simulink model "main"  (R2025b)
settings: Solver=FixedStepDiscrete  StartTime=0.0  StopTime=Inf  RelTol=1e-3  EnableMultiTasking=on
PreLoadFcn:
  | RTWConfigurationCB('preloadfcn', bdroot);
model workspace (MAT data in the model file):
  fault_count = 0
  fz_values = [0 50 100 150 200 250 300 350 400 450 500 550 ... (43 elements, 1x43)]
  k_opt_lut = [0 0 0 0 0 0 0 0 0 0 0 0 ... (4386 elements, 51x2x43)]
  mu_opt_lut = [0 0 0 0 0 0 0 0 0 0 0 0 ... (4386 elements, 51x2x43)]
undefined symbols (not defined in the file or in its folder): bit, Call, Function, ocv_lut, slope_lut, soc_lut
libraries: c2837xDlib x34, c280xlib x20, canmsglib x18, c2802xlib x12, simulink x9, slpidlib x3
(part 3 of 5)

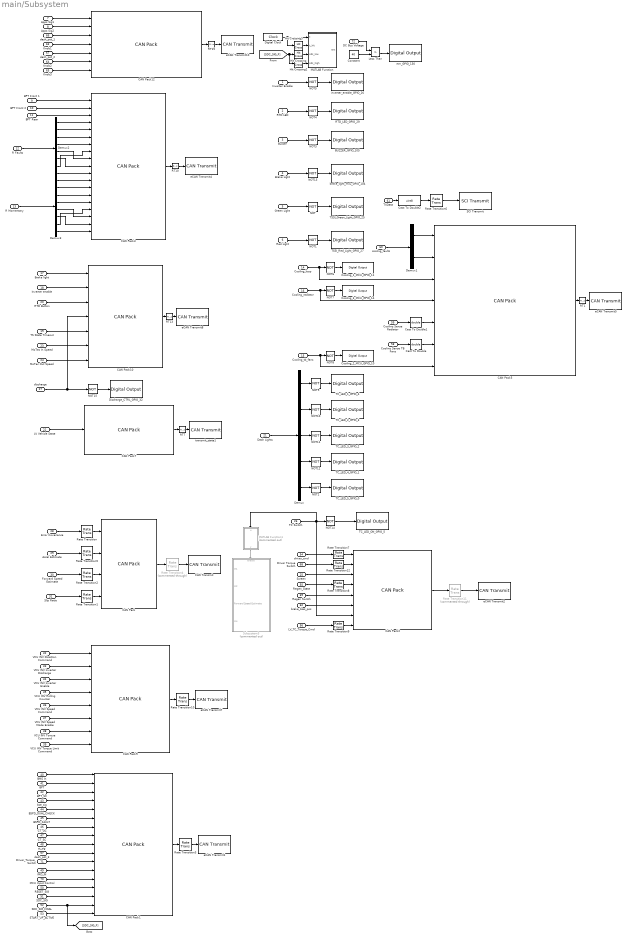
== system main/Subsystem ==
  Inverter Enable : Inport
  RTD LED : Inport  Port=2
  Buzzer : Inport  Port=3
  Brake Light : Inport  Port=4
  Green Light : Inport  Port=5
  Red Light : Inport  Port=6
  Apps Sig1 : Inport  Port=7
  Apps Sig2 : Inport  Port=8
  BPT Front 1 : Inport  Port=9
  BPT Front 2 : Inport  Port=10
  BPT Rear : Inport  Port=11
  R Faults : Inport  Port=12
  R Momentary : Inport  Port=13
  Cooling_loop : Inport  Port=14
  Cooling_tb_fans : Inport  Port=15
  Cooling_radiator : Inport  Port=16
  Brake light : Inport  Port=17
  Inverter enable : Inport  Port=18
  TS State Timeout : Inport  Port=19
  RTD Button : Inport  Port=20
  Dash Lights : Inport  Port=21
  LV Vehicle State : Inport  Port=22
  MoTec In Speed : Inport  Port=23
  MoTec Out Speed : Inport  Port=24
  Screen : Inport  Port=25
  TC Switch : Inport  Port=26
  discharge : Inport  Port=27
  Error Covariance : Inport  Port=28
  Accel Estimate : Inport  Port=29
  Forward Speed Estimate : Inport  Port=30
  Slip Ratio : Inport  Port=31
  VCU INV Direction Command : Inport  Port=32
  VCU INV Inverter Discharge : Inport  Port=33
  VCU INV Inverter Enable : Inport  Port=34
  VCU INV Rolling Counter : Inport  Port=35
  VCU INV Speed Command : Inport  Port=36
  VCU INV Speed Mode Enable : Inport  Port=37
  VCU INV Torque Command : Inport  Port=38
  VCU INV Torque Limit Command : Inport  Port=39
  BMS In : Inport  Port=40
  BPT : Inport  Port=41
  BPT_SC : Inport  Port=42
  bse_sig : Inport  Port=43
  BSPD_DUAL_CHECK : Inport  Port=44
  BSPD_FAULT : Inport  Port=45
  CT_OC : Inport  Port=46
  CT_SC : Inport  Port=47
  ct_sig : Inport  Port=48
  IMD_IN : Inport  Port=49
  RESET_SIG : Inport  Port=50
  SDC_SIG : Inport  Port=51
  SDC_SIG_FINAL : Inport  Port=52
  START_UP_ACTIVE : Inport  Port=53
  driver_cmd : Inport  Port=54
  Regen_State : Inport  Port=55
  LV_TC_Torque_Cmd : Inport  Port=56
  dash_pot_3 : Inport  Port=57
  Cooling Sense TB Fans : Inport  Port=58
  Cooling Sense Radiator : Inport  Port=59
  cooling_faults : Inport  Port=60
  TXData : Inport  Port=61
  brake_bias_pos : Inport  Port=62
  Knob1 : Inport  Port=63
  Knob2 : Inport  Port=64
  Knob3 : Inport  Port=65
  dash_pot_1 : Inport  Port=66
  dash_pot_2 : Inport  Port=67
  Driver Torque Switch : Inport  Port=68
  Regen Switch : Inport  Port=69
  MCU Input Control : Inport  Port=70
  Driver_Torque_Switch : Inport  Port=71
  DC Bus Voltage : Inport  Port=72
  BUZZER_GPIO_105 : c2837xDlib/Digital Output  GPIO_Number=GPIO104~GPIO111  GPIO_Bit0=off  GPIO_BIT0_Toggle=off  GPIO_Bit1=on  GPIO_BIT1_Toggle=off  GPIO_Bit2=off  GPIO_BIT2_Toggle=off  GPIO_Bit3=off  GPIO_BIT3_Toggle=off  GPIO_Bit4=off  GPIO_BIT4_Toggle=off  GPIO_Bit5=off  GPIO_BIT5_Toggle=off  GPIO_Bit6=off  GPIO_BIT6_Toggle=off  GPIO_Bit7=off  GPIO_BIT7_Toggle=off
  CAN Pack : canmsglib/CAN Pack  CANdbFile=C:\Users\Columbia\Documents\GitHub\EV26-Software\CAN\EV26.dbc  MsgList=(none)  MsgName=M404_LV_V_Kalman_Outputs  MsgIDType=Standard (11-bit identifier)  MsgIdentifier=404  CANIDInput=off  MsgLength=8  Remote=off  ApplyMinMax=off  BusOutput=off  SignalInfo={'LV_COV_V','32','16','LE','unsigned','Standard','0','0.02','0','0','1310.7';'LV_FILTERED_A','16','16','LE','signed','Standard','0','0.01','0','-327.68','327.67';'LV_FILTERED_V','0','16','LE','unsigned','Standard','0','0.1','0','0','6553.5';'LV_SR','48','16','LE','signed','Standard','0','0.0001','0','-3.2768','3.2767'}
      settings: LibrarySourceBlock=c2000lib/Target Communication/CAN Pack  DataFormat=CANdb specified signals
  CAN Pack1 : canmsglib/CAN Pack  CANdbFile=C:\Users\levin\OneDrive\Documents\GitHub\EV26-Software\CAN\EV26.dbc  MsgList=M406_Board_Signals  MsgName=M406_Board_Signals  MsgIDType=Standard (11-bit identifier)  MsgIdentifier=406  CANIDInput=off  MsgLength=8  Remote=off  ApplyMinMax=off  BusOutput=off  SignalInfo={'LV_BMS_Good','1','1','LE','unsigned','Standard','0','1','0','0','1';'LV_BPT_OC','3','1','LE','unsigned','Standard','0','1','0','0','1';'LV_BPT_SC','2','1','LE','unsigned','Standard','0','1','0','0','1';'LV_BSE_Sig','16','16','LE','signed','Standard','0','1','0','-32768','32767';'LV_BSPD_Dual_Check','6','1','LE','unsigned','Standard','0','1','0','0','1';'LV_BSPD_Fault','7','1','LE','unsigned','Standard','0','1','0','0','1';'LV_CT_OC','5','1','LE','unsigned','Standard','0','1','0','0','1';'LV_CT_SC','4','1','LE','unsigned','Standard','0','1','0','0','1';'LV_CT_Sig','32','16','LE','signed','Standard','0','1','0','-32768','32767';'LV_Dash_Pot_3','48','8','LE','unsigned','Standard','0','20','0','0','5100';'LV_Driver_Torque_Switch','56','1','LE','unsigned','Standard','0','1','0','0','1';'LV_IMD_Good','0','1','LE','unsigned','Standard','0','1','0','0','1';'LV_MCU_Torque_Ctrl','12','3','LE','unsigned','Standard','0','1','0','0','7';'LV_Reset_Sig','10','1','LE','unsigned','Standard','0','1','0','0','1';'LV_SDC_Sig','11','1','LE','unsigned','Standard','0','1','0','0','1';'LV_SDC_Sig_Final','9','1','LE','unsigned','Standard','0','1','0','0','1';'LV_Start_Up_Active','8','1','LE','unsigned','Standard','0','1','0','0','1'}
      settings: DataFormat=CANdb specified signals
  CAN Pack10 : canmsglib/CAN Pack  CANdbFile=C:\Users\levin\OneDrive\Documents\GitHub\EV26-Software\CAN\EV26.dbc  MsgList=M403_Vehicle_State_Inputs  MsgName=M403_Vehicle_State_Inputs  MsgIDType=Standard (11-bit identifier)  MsgIdentifier=403  CANIDInput=off  MsgLength=8  Remote=off  ApplyMinMax=off  BusOutput=off  SignalInfo={'LV_Brake_Light','0','8','LE','unsigned','Standard','0','1','0','-Inf','Inf';'LV_Echo_Inverter_Enable','8','8','LE','signed','Standard','0','1','0','-Inf','Inf';'LV_RTD_Button','24','8','LE','unsigned','Standard','0','1','0','-Inf','Inf';'LV_TB_Discharge','32','1','LE','unsigned','Standard','0','1','0','0','1';'LV_TB_TS_State_Timeout','16','8','LE','signed','Standard','0','1','0','-Inf','Inf';'MoTec_In_Speed','40','12','LE','unsigned','Standard','0','0.1','0','0','409.5';'MoTec_Out_Speed','52','12','LE','unsigned','Standard','0','0.1','0','0','409.5'}
      settings: DataFormat=CANdb specified signals
  CAN Pack12 : canmsglib/CAN Pack  CANdbFile=C:\Users\levin\OneDrive\Documents\GitHub\EV26-Software\CAN\EV26.dbc  MsgList=M401_Accelerator_Controls  MsgName=M401_Accelerator_Controls  MsgIDType=Standard (11-bit identifier)  MsgIdentifier=401  CANIDInput=off  MsgLength=8  Remote=off  ApplyMinMax=off  BusOutput=off  SignalInfo={'LV_APPS1','0','16','LE','unsigned','Standard','0','1','0','0','4095';'LV_APPS2','16','16','LE','unsigned','Standard','0','1','0','0','4095';'LV_Dash_Pot_1','44','8','LE','unsigned','Standard','0','20','0','0','5100';'LV_Dash_Pot_1_Tick','32','4','LE','unsigned','Standard','0','1','0','0','15';'LV_Dash_Pot_2','52','8','LE','unsigned','Standard','0','20','0','0','5100';'LV_Dash_Pot_2_Tick','36','4','LE','unsigned','Standard','0','1','0','0','15';'LV_Dash_Pot_3_Tick','40','4','LE','unsigned','Standard','0','1','0','0','15'}
      settings: DataFormat=CANdb specified signals
  CAN Pack2 : canmsglib/CAN Pack  CANdbFile=C:\Users\levin\OneDrive\Documents\GitHub\EV26-Software\CAN\EV26.dbc  MsgList=M405_TC_Regen_Signals  MsgName=M405_TC_Regen_Signals  MsgIDType=Standard (11-bit identifier)  MsgIdentifier=405  CANIDInput=off  MsgLength=8  Remote=off  ApplyMinMax=off  BusOutput=off  SignalInfo={'LV_Driver_Torque','16','16','LE','signed','Standard','0','0.1','0','-3276.8','3276.7';'LV_Driver_Torque_Switch','58','1','LE','unsigned','Standard','0','1','0','0','1';'LV_MoTec_Screen','48','8','LE','unsigned','Standard','0','1','0','0','255';'LV_Regen_State','32','8','LE','signed','Standard','0','1','0','-128','127';'LV_Regen_Switch','57','1','LE','unsigned','Standard','0','1','0','0','1';'LV_Servo_Pos','40','8','LE','signed','Standard','0','160.6275','0','-20560.3137','20399.6863';'LV_TC_Switch','56','1','LE','unsigned','Standard','0','1','0','0','1';'LV_TC_Torque_Cmd','0','16','LE','signed','Standard','0','0.1','0','-3276.8','3276.7'}
      settings: DataFormat=CANdb specified signals
  CAN Pack3 : canmsglib/CAN Pack  CANdbFile=C:\Users\Columbia\Documents\GitHub\EV26-Software\CAN\EV26.dbc  MsgList=(none)  MsgName=M402_Brakes_Faults_Display  MsgIDType=Standard (11-bit identifier)  MsgIdentifier=402  CANIDInput=off  MsgLength=8  Remote=off  ApplyMinMax=off  BusOutput=off  SignalInfo={'LV_BPT_Front_1','16','16','LE','unsigned','Standard','0','1','0','-Inf','Inf';'LV_BPT_Front_2','32','16','LE','unsigned','Standard','0','1','0','-Inf','Inf';'LV_BPT_Rear','0','16','LE','unsigned','Standard','0','1','0','-Inf','Inf';'LV_Fault_APPS1_Lower','48','1','LE','unsigned','Standard','0','1','0','0','1';'LV_Fault_APPS1_Upper','49','1','LE','unsigned','Standard','0','1','0','0','1';'LV_Fault_APPS2_Lower','50','1','LE','unsigned','Standard','0','1','0','0','1';'LV_Fault_APPS2_Upper','51','1','LE','unsigned','Standard','0','1','0','0','1';'LV_Fault_APPS_Implausibility','54','1','LE','unsigned','Standard','0','1','0','0','1';'LV_Fault_BPT_Lower','52','1','LE','unsigned','Standard','0','1','0','0','1';'LV_Fault_BPT_Upper','53','1','LE','unsigned','Standard','0','1','0','0','1';'LV_Fault_Both_Pedals','55','1','LE','unsigned','Standard','0','1','0','0','1';'LV_Momentary_APPS1_Lower','56','1','LE','unsigned','Standard','0','1','0','0','1';'LV_Momentary_APPS1_Upper','57','1','LE','unsigned','Standard','0','1','0','0','1';'LV_Momentary_APPS2_Lower','58','1','LE','unsigned','Standard','0','1','0','0','1';'LV_Momentary_APPS2_Upper','59','1','LE','unsigned','Standard','0','1','0','0','1';'LV_Momentary_APPS_Implausibility','62','1','LE','unsigned','Standard','0','1','0','0','1';'LV_Momentary_BPT_Lower','60','1','LE','unsigned','Standard','0','1','0','0','1';'LV_Momentary_BPT_Upper','61','1','LE','unsigned','Standard','0','1','0','0','1';'LV_Momentary_Both_Pedals','63','1','LE','unsigned','Standard','0','1','0','0','1'}
      settings: DataFormat=CANdb specified signals
  CAN Pack5 : canmsglib/CAN Pack  CANdbFile=C:\Users\levin\OneDrive\Documents\GitHub\EV26-Software\CAN\EV26.dbc  MsgList=M003_DCDC_Enable_Cooling  MsgName=M003_DCDC_Enable_Cooling  MsgIDType=Standard (11-bit identifier)  MsgIdentifier=3  CANIDInput=off  MsgLength=8  Remote=off  ApplyMinMax=off  BusOutput=off  SignalInfo={'LV_TB_Cooling_Fault_Radiator','36','1','LE','unsigned','Standard','0','1','0','0','1';'LV_TB_Cooling_Fault_TB_Fans','35','1','LE','unsigned','Standard','0','1','0','0','1';'LV_TB_Cooling_Loop','32','1','LE','unsigned','Standard','0','1','0','0','1';'LV_TB_Cooling_Radiator','34','1','LE','unsigned','Standard','0','1','0','0','1';'LV_TB_Cooling_Sense_Radiator','16','16','LE','signed','Standard','0','0.01','0','-327.68','327.67';'LV_TB_Cooling_Sense_TB_Fans','0','16','LE','signed','Standard','0','0.01','0','-327.68','327.67';'LV_TB_Cooling_TB_Fans','33','1','LE','unsigned','Standard','0','1','0','0','1'}
      settings: DataFormat=CANdb specified signals
  CAN Pack7 : canmsglib/CAN Pack  CANdbFile=C:\Users\Columbia\Documents\GitHub\EV26-Software\CAN\EV26.dbc  MsgList=(none)  MsgName=M001_Vehicle_State  MsgIDType=Standard (11-bit identifier)  MsgIdentifier=1  CANIDInput=off  MsgLength=1  Remote=off  ApplyMinMax=off  BusOutput=off  SignalInfo={'LV_Vehicle_State','0','8','LE','signed','Standard','0','1','0','-Inf','Inf'}
      settings: DataFormat=CANdb specified signals
  CAN Pack9 : canmsglib/CAN Pack  CANdbFile=C:\Users\levin\OneDrive\Documents\GitHub\EV26-Software\CAN\EV26.dbc  MsgList=M192_Command_Message  MsgName=M192_Command_Message  MsgIDType=Standard (11-bit identifier)  MsgIdentifier=192  CANIDInput=off  MsgLength=8  Remote=off  ApplyMinMax=off  BusOutput=off  SignalInfo={'VCU_INV_Direction_Command','32','1','LE','unsigned','Standard','0','1','0','0','1';'VCU_INV_Inverter_Discharge','41','1','LE','unsigned','Standard','0','1','0','0','1';'VCU_INV_Inverter_Enable','40','1','LE','unsigned','Standard','0','1','0','0','1';'VCU_INV_Rolling_Counter','44','4','LE','unsigned','Standard','0','1','0','0','15';'VCU_INV_Speed_Command','16','16','LE','signed','Standard','0','1','0','-32768','32767';'VCU_INV_Speed_Mode_Enable','42','1','LE','unsigned','Standard','0','1','0','0','1';'VCU_INV_Torque_Command','0','16','LE','signed','Standard','0','0.1','0','-3276.8','3276.7';'VCU_INV_Torque_Limit_Command','48','16','LE','signed','Standard','0','0.1','0','-3276.8','3276.7'}
      settings: DataFormat=CANdb specified signals
  CAN Transmit : c280xlib/CAN Transmit  chipFamily=C280x  useModule=CAN_B  mailboxNo=11  messageID=404  messageType=Standard (11-bit identifier)  enableBlockingMode=off  postInterrupt=off  interruptLine=0
  Cast To Double : DataTypeConversion  OutDataTypeStr=double  SaturateOnIntegerOverflow=off  RndMeth=Floor
  Cast To Double1 : DataTypeConversion  OutDataTypeStr=double  SaturateOnIntegerOverflow=off  RndMeth=Floor
  Cast To Double2 : DataTypeConversion  OutDataTypeStr=uint8  SaturateOnIntegerOverflow=off  RndMeth=Floor
  Constant : Constant  Value=40
  Cooling_1_MCU_GPIO_11 : c2837xDlib/Digital Output  GPIO_Number=GPIO8~GPIO15  GPIO_Bit0=off  GPIO_BIT0_Toggle=off  GPIO_Bit1=off  GPIO_BIT1_Toggle=off  GPIO_Bit2=off  GPIO_BIT2_Toggle=off  GPIO_Bit3=on  GPIO_BIT3_Toggle=off  GPIO_Bit4=off  GPIO_BIT4_Toggle=off  GPIO_Bit5=off  GPIO_BIT5_Toggle=off  GPIO_Bit6=off  GPIO_BIT6_Toggle=off  GPIO_Bit7=off  GPIO_BIT7_Toggle=off
  Cooling_2_MCU_GPIO_10 : c2837xDlib/Digital Output  GPIO_Number=GPIO8~GPIO15  GPIO_Bit0=off  GPIO_BIT0_Toggle=off  GPIO_Bit1=off  GPIO_BIT1_Toggle=off  GPIO_Bit2=on  GPIO_BIT2_Toggle=off  GPIO_Bit3=off  GPIO_BIT3_Toggle=off  GPIO_Bit4=off  GPIO_BIT4_Toggle=off  GPIO_Bit5=off  GPIO_BIT5_Toggle=off  GPIO_Bit6=off  GPIO_BIT6_Toggle=off  GPIO_Bit7=off  GPIO_BIT7_Toggle=off
  Cooling_3_MCU_GPIO_14 : c2837xDlib/Digital Output  GPIO_Number=GPIO8~GPIO15  GPIO_Bit0=off  GPIO_BIT0_Toggle=off  GPIO_Bit1=off  GPIO_BIT1_Toggle=off  GPIO_Bit2=off  GPIO_BIT2_Toggle=off  GPIO_Bit3=off  GPIO_BIT3_Toggle=off  GPIO_Bit4=off  GPIO_BIT4_Toggle=off  GPIO_Bit5=off  GPIO_BIT5_Toggle=off  GPIO_Bit6=on  GPIO_BIT6_Toggle=off  GPIO_Bit7=off  GPIO_BIT7_Toggle=off
  Demux : Demux  Outputs=5
  Demux1 : Demux  Outputs=2
  Demux2 : Demux  Outputs=8
  Demux3 : Demux  Outputs=8
  Digital Clock : DigitalClock  SampleTime=0.001
  Discharge_CTRL_GPIO_32 : c2837xDlib/Digital Output  GPIO_Number=GPIO32~GPIO39  GPIO_Bit0=on  GPIO_BIT0_Toggle=off  GPIO_Bit1=off  GPIO_BIT1_Toggle=off  GPIO_Bit2=off  GPIO_BIT2_Toggle=off  GPIO_Bit3=off  GPIO_BIT3_Toggle=off  GPIO_Bit4=off  GPIO_BIT4_Toggle=off  GPIO_Bit5=off  GPIO_BIT5_Toggle=off  GPIO_Bit6=off  GPIO_BIT6_Toggle=off  GPIO_Bit7=off  GPIO_BIT7_Toggle=off
  Hit Crossing : HitCross  HitCrossingDirection=falling
  Hit Crossing2 : HitCross  HitCrossingOffset=1  HitCrossingDirection=rising
  Hit Crossing3 : HitCross  HitCrossingOffset=4  HitCrossingDirection=rising
  Less Than : RelationalOperator  Operator=>  OutDataTypeStr=boolean  RndMeth=Simplest  InputSameDT=off
  MATLAB Function : MATLAB Function  TreatAsAtomicUnit=on
  MATLAB Function1 : MATLAB Function  Commented=on  TreatAsAtomicUnit=on
  NOT{,1..15} (16 alike) : Logic  Operator=NOT  IconShape=distinctive  AllPortsSameDT=off  OutDataTypeStr=boolean
  RT1 : RateTransition  OutPortSampleTime=.1
  RT10 : RateTransition  OutPortSampleTime=.01
  RT13 : RateTransition  OutPortSampleTime=.05
  RT15 : RateTransition  OutPortSampleTime=0.01
  RT7 : RateTransition  OutPortSampleTime=.1
  RTD_LED_GPIO_29 : c2837xDlib/Digital Output  GPIO_Number=GPIO24~GPIO31  GPIO_Bit0=off  GPIO_BIT0_Toggle=off  GPIO_Bit1=off  GPIO_BIT1_Toggle=off  GPIO_Bit2=off  GPIO_BIT2_Toggle=off  GPIO_Bit3=off  GPIO_BIT3_Toggle=off  GPIO_Bit4=off  GPIO_BIT4_Toggle=off  GPIO_Bit5=on  GPIO_BIT5_Toggle=off  GPIO_Bit6=off  GPIO_BIT6_Toggle=off  GPIO_Bit7=off  GPIO_BIT7_Toggle=off
  Rate Transition{,1..3,5,7..9,12} (9 alike) : RateTransition  OutPortSampleTime=0.01
  Rate Transition10 : RateTransition  OutPortSampleTime=0.003
  Rate Transition11 : RateTransition  Commented=through  OutPortSampleTime=0.003
  Rate Transition4 : RateTransition  Commented=through  OutPortSampleTime=0.05
  Rate Transition6 : RateTransition  OutPortSampleTime=1
  SCI Transmit : c280xlib/SCI Transmit  sciModule=C  dataHead='S'  dataTail='E'  frameSize=1  blockingMode=on  outputStatus=off
      settings: LibrarySourceBlock=c2802xlib/SCI Transmit
  Subsystem3 : Subsystem  Commented=on
  TC_LED_1_GPIO_4 : c2837xDlib/Digital Output  GPIO_Number=GPIO0~GPIO7  GPIO_Bit0=off  GPIO_BIT0_Toggle=off  GPIO_Bit1=off  GPIO_BIT1_Toggle=off  GPIO_Bit2=off  GPIO_BIT2_Toggle=off  GPIO_Bit3=off  GPIO_BIT3_Toggle=off  GPIO_Bit4=on  GPIO_BIT4_Toggle=off  GPIO_Bit5=off  GPIO_BIT5_Toggle=off  GPIO_Bit6=off  GPIO_BIT6_Toggle=off  GPIO_Bit7=off  GPIO_BIT7_Toggle=off
  TC_LED_2_GPIO_3 : c2837xDlib/Digital Output  GPIO_Number=GPIO0~GPIO7  GPIO_Bit0=off  GPIO_BIT0_Toggle=off  GPIO_Bit1=off  GPIO_BIT1_Toggle=off  GPIO_Bit2=off  GPIO_BIT2_Toggle=off  GPIO_Bit3=on  GPIO_BIT3_Toggle=off  GPIO_Bit4=off  GPIO_BIT4_Toggle=off  GPIO_Bit5=off  GPIO_BIT5_Toggle=off  GPIO_Bit6=off  GPIO_BIT6_Toggle=off  GPIO_Bit7=off  GPIO_BIT7_Toggle=off
  TC_LED_3_GPIO_2 : c2837xDlib/Digital Output  GPIO_Number=GPIO0~GPIO7  GPIO_Bit0=off  GPIO_BIT0_Toggle=off  GPIO_Bit1=off  GPIO_BIT1_Toggle=off  GPIO_Bit2=on  GPIO_BIT2_Toggle=off  GPIO_Bit3=off  GPIO_BIT3_Toggle=off  GPIO_Bit4=off  GPIO_BIT4_Toggle=off  GPIO_Bit5=off  GPIO_BIT5_Toggle=off  GPIO_Bit6=off  GPIO_BIT6_Toggle=off  GPIO_Bit7=off  GPIO_BIT7_Toggle=off
  TC_LED_4_GPIO_1 : c2837xDlib/Digital Output  GPIO_Number=GPIO0~GPIO7  GPIO_Bit0=off  GPIO_BIT0_Toggle=off  GPIO_Bit1=on  GPIO_BIT1_Toggle=off  GPIO_Bit2=off  GPIO_BIT2_Toggle=off  GPIO_Bit3=off  GPIO_BIT3_Toggle=off  GPIO_Bit4=off  GPIO_BIT4_Toggle=off  GPIO_Bit5=off  GPIO_BIT5_Toggle=off  GPIO_Bit6=off  GPIO_BIT6_Toggle=off  GPIO_Bit7=off  GPIO_BIT7_Toggle=off
  TC_LED_5_GPIO_0 : c2837xDlib/Digital Output  GPIO_Number=GPIO0~GPIO7  GPIO_Bit0=on  GPIO_BIT0_Toggle=off  GPIO_Bit1=off  GPIO_BIT1_Toggle=off  GPIO_Bit2=off  GPIO_BIT2_Toggle=off  GPIO_Bit3=off  GPIO_BIT3_Toggle=off  GPIO_Bit4=off  GPIO_BIT4_Toggle=off  GPIO_Bit5=off  GPIO_BIT5_Toggle=off  GPIO_Bit6=off  GPIO_BIT6_Toggle=off  GPIO_Bit7=off  GPIO_BIT7_Toggle=off
  TC_LED_ON_GPIO_5 : c2837xDlib/Digital Output  GPIO_Number=GPIO0~GPIO7  GPIO_Bit0=off  GPIO_BIT0_Toggle=off  GPIO_Bit1=off  GPIO_BIT1_Toggle=off  GPIO_Bit2=off  GPIO_BIT2_Toggle=off  GPIO_Bit3=off  GPIO_BIT3_Toggle=off  GPIO_Bit4=off  GPIO_BIT4_Toggle=off  GPIO_Bit5=on  GPIO_BIT5_Toggle=off  GPIO_Bit6=off  GPIO_BIT6_Toggle=off  GPIO_Bit7=off  GPIO_BIT7_Toggle=off
  TSSI_Green_Light_GPIO_25 : c2837xDlib/Digital Output  GPIO_Number=GPIO24~GPIO31  GPIO_Bit0=off  GPIO_BIT0_Toggle=off  GPIO_Bit1=on  GPIO_BIT1_Toggle=off  GPIO_Bit2=off  GPIO_BIT2_Toggle=off  GPIO_Bit3=off  GPIO_BIT3_Toggle=off  GPIO_Bit4=off  GPIO_BIT4_Toggle=off  GPIO_Bit5=off  GPIO_BIT5_Toggle=off  GPIO_Bit6=off  GPIO_BIT6_Toggle=off  GPIO_Bit7=off  GPIO_BIT7_Toggle=off
  TSSI_Red_Light_GPIO_27 : c2837xDlib/Digital Output  GPIO_Number=GPIO24~GPIO31  GPIO_Bit0=off  GPIO_BIT0_Toggle=off  GPIO_Bit1=off  GPIO_BIT1_Toggle=off  GPIO_Bit2=off  GPIO_BIT2_Toggle=off  GPIO_Bit3=on  GPIO_BIT3_Toggle=off  GPIO_Bit4=off  GPIO_BIT4_Toggle=off  GPIO_Bit5=off  GPIO_BIT5_Toggle=off  GPIO_Bit6=off  GPIO_BIT6_Toggle=off  GPIO_Bit7=off  GPIO_BIT7_Toggle=off
  brake_light_mcu_GPIO_104 : c2837xDlib/Digital Output  GPIO_Number=GPIO104~GPIO111  GPIO_Bit0=on  GPIO_BIT0_Toggle=off  GPIO_Bit1=off  GPIO_BIT1_Toggle=off  GPIO_Bit2=off  GPIO_BIT2_Toggle=off  GPIO_Bit3=off  GPIO_BIT3_Toggle=off  GPIO_Bit4=off  GPIO_BIT4_Toggle=off  GPIO_Bit5=off  GPIO_BIT5_Toggle=off  GPIO_Bit6=off  GPIO_BIT6_Toggle=off  GPIO_Bit7=off  GPIO_BIT7_Toggle=off
  eCAN Transmit1 : c280xlib/CAN Transmit  chipFamily=C280x  useModule=CAN_B  mailboxNo=16  messageID=192  messageType=Standard (11-bit identifier)  enableBlockingMode=off  postInterrupt=off  interruptLine=0
  eCAN Transmit10 : c280xlib/CAN Transmit  chipFamily=C280x  useModule=CAN_B  mailboxNo=6  messageID=401  messageType=Standard (11-bit identifier)  enableBlockingMode=off  postInterrupt=off  interruptLine=0
  eCAN Transmit2 : c280xlib/CAN Transmit  chipFamily=C280x  useModule=CAN_B  mailboxNo=17  messageID=192  messageType=Standard (11-bit identifier)  enableBlockingMode=off  postInterrupt=off  interruptLine=0
  eCAN Transmit4 : c280xlib/CAN Transmit  chipFamily=C280x  useModule=CAN_B  mailboxNo=7  messageID=402  messageType=Standard (11-bit identifier)  enableBlockingMode=off  postInterrupt=off  interruptLine=0
  eCAN Transmit5 : c280xlib/CAN Transmit  chipFamily=C280x  useModule=CAN_B  mailboxNo=18  messageID=403  messageType=Standard (11-bit identifier)  enableBlockingMode=off  postInterrupt=off  interruptLine=0
  eCAN Transmit7 : c280xlib/CAN Transmit  chipFamily=C280x  useModule=CAN_B  mailboxNo=4  messageID=192  messageType=Standard (11-bit identifier)  enableBlockingMode=off  postInterrupt=off  interruptLine=0
  eCAN Transmit8 : c280xlib/CAN Transmit  chipFamily=C280x  useModule=CAN_B  mailboxNo=8  messageID=403  messageType=Standard (11-bit identifier)  enableBlockingMode=off  postInterrupt=off  interruptLine=0
  inverter_enable_GPIO_26 : c2837xDlib/Digital Output  GPIO_Number=GPIO24~GPIO31  GPIO_Bit0=off  GPIO_BIT0_Toggle=off  GPIO_Bit1=off  GPIO_BIT1_Toggle=off  GPIO_Bit2=on  GPIO_BIT2_Toggle=off  GPIO_Bit3=off  GPIO_BIT3_Toggle=off  GPIO_Bit4=off  GPIO_BIT4_Toggle=off  GPIO_Bit5=off  GPIO_BIT5_Toggle=off  GPIO_Bit6=off  GPIO_BIT6_Toggle=off  GPIO_Bit7=off  GPIO_BIT7_Toggle=off
  rtm_GPIO_130 : c2837xDlib/Digital Output  GPIO_Number=GPIO128~GPIO135  GPIO_Bit0=off  GPIO_BIT0_Toggle=off  GPIO_Bit1=off  GPIO_BIT1_Toggle=off  GPIO_Bit2=on  GPIO_BIT2_Toggle=off  GPIO_Bit3=off  GPIO_BIT3_Toggle=off  GPIO_Bit4=off  GPIO_BIT4_Toggle=off  GPIO_Bit5=off  GPIO_BIT5_Toggle=off  GPIO_Bit6=off  GPIO_BIT6_Toggle=off  GPIO_Bit7=off  GPIO_BIT7_Toggle=off
  transmit_state1 : c280xlib/CAN Transmit  chipFamily=C280x  useModule=CAN_B  mailboxNo=1  messageID=1  messageType=Standard (11-bit identifier)  enableBlockingMode=off  postInterrupt=off  interruptLine=0
  wires:
  Demux2/7 -> CAN Pack3/8
  Error Covariance/1 -> Rate Transition/1
  MATLAB Function1/1(y) -> Subsystem3/Enable
  Demux/3 -> NOT11/1
  Demux3/3 -> CAN Pack3/14
  RT13/1 -> eCAN Transmit8/1
  CAN Pack7/1 -> RT7/1
  Green Light/1 -> NOT/1
  CAN Pack12/1 -> RT15/1
  MoTec Out Speed/1 -> CAN Pack10/7
  Demux3/7 -> CAN Pack3/16
  ct_sig/1 -> CAN Pack1/9
  Rate Transition10/1 -> eCAN Transmit7/1
  VCU INV Direction Command/1 -> CAN Pack9/1
  Demux/4 -> NOT12/1
  Cooling_tb_fans/1 -> CAN Pack5/7, NOT8/1
  CAN Pack9/1 -> Rate Transition10/1
  Demux3/6 -> CAN Pack3/18
  Demux/1 -> NOT9/1
  Demux3/5 -> CAN Pack3/17
  Demux/2 -> NOT10/1
  RTD Button/1 -> CAN Pack10/3
  RT7/1 -> transmit_state1/1
  Demux2/5 -> CAN Pack3/9
  Demux3/2 -> CAN Pack3/13
  RT15/1 -> eCAN Transmit10/1
  VCU INV Speed Mode Enable/1 -> CAN Pack9/6
  CAN Pack1/1 -> Rate Transition3/1
  VCU INV Speed Command/1 -> CAN Pack9/5
  Demux2/3 -> CAN Pack3/6
  RT10/1 -> eCAN Transmit4/1
  Demux3/4 -> CAN Pack3/15
  Demux2/4 -> CAN Pack3/7
  Demux3/8 -> CAN Pack3/19
  Dash Lights/1 -> Demux/1
  Demux2/2 -> CAN Pack3/5
  R Momentary/1 -> Demux3/1
  VCU INV Inverter Enable/1 -> CAN Pack9/3
  Demux2/6 -> CAN Pack3/10
  CAN Pack2/1 -> Rate Transition11/1
  BPT/1 -> CAN Pack1/2
  VCU INV Inverter Discharge/1 -> CAN Pack9/2
  Demux2/8 -> CAN Pack3/11
  Demux2/1 -> CAN Pack3/4
  BSPD_DUAL_CHECK/1 -> CAN Pack1/5
  CAN Pack3/1 -> RT10/1
  Rate Transition11/1 -> eCAN Transmit2/1
  Cooling_radiator/1 -> CAN Pack5/4, NOT7/1
  Demux3/1 -> CAN Pack3/12
  driver_cmd/1 -> Rate Transition7/1
  CAN Pack10/1 -> RT13/1
  Slip Ratio/1 -> Rate Transition1/1
  MoTec In Speed/1 -> CAN Pack10/6
  BPT Front 1/1 -> CAN Pack3/1
  BPT Rear/1 -> CAN Pack3/3
  bse_sig/1 -> CAN Pack1/4
  RTD LED/1 -> NOT4/1
  Inverter Enable/1 -> NOT5/1
  LV_TC_Torque_Cmd/1 -> Rate Transition9/1
  BSPD_FAULT/1 -> CAN Pack1/6
  Accel Estimate/1 -> Rate Transition5/1
  LV Vehicle State/1 -> CAN Pack7/1
  Apps Sig1/1 -> CAN Pack12/1
  Red Light/1 -> NOT1/1
  VCU INV Rolling Counter/1 -> CAN Pack9/4
  Apps Sig2/1 -> CAN Pack12/2
  Regen_State/1 -> Rate Transition8/1
  Inverter enable/1 -> CAN Pack10/2
  TS State Timeout/1 -> CAN Pack10/5
  CT_OC/1 -> CAN Pack1/7
  VCU INV Torque Limit Command/1 -> CAN Pack9/8
  VCU INV Torque Command/1 -> CAN Pack9/7
  Screen/1 -> CAN Pack2/3
  TC Switch/1 -> CAN Pack2/7, NOT14/1, MATLAB Function1/1(u)
  BPT_SC/1 -> CAN Pack1/3
  CT_SC/1 -> CAN Pack1/8
  Forward Speed Estimate/1 -> Rate Transition2/1
  BMS In/1 -> CAN Pack1/1
  Brake light/1 -> CAN Pack10/1
  R Faults/1 -> Demux2/1
  Cooling_loop/1 -> CAN Pack5/3, NOT6/1
  RT1/1 -> eCAN Transmit5/1
  CAN Pack5/1 -> RT1/1
  Cooling Sense TB Fans/1 -> Cast To Double/1
  Cooling Sense Radiator/1 -> Cast To Double1/1
  cooling_faults/1 -> Demux1/1
  Cast To Double1/1 -> CAN Pack5/5
  BPT Front 2/1 -> CAN Pack3/2
  Demux1/1 -> CAN Pack5/1
  Demux1/2 -> CAN Pack5/2
  Cast To Double/1 -> CAN Pack5/6
  Rate Transition/1 -> CAN Pack/1
  Rate Transition5/1 -> CAN Pack/2
  Rate Transition2/1 -> CAN Pack/3
  Rate Transition1/1 -> CAN Pack/4
  discharge/1 -> NOT15/1, CAN Pack10/4
  TXData/1 -> Cast To Double2/1
  Cast To Double2/1 -> Rate Transition6/1
  Rate Transition6/1 -> SCI Transmit/1
  brake_bias_pos/1 -> CAN Pack2/6
  Rate Transition7/1 -> CAN Pack2/1
  Rate Transition8/1 -> CAN Pack2/4
  Rate Transition9/1 -> CAN Pack2/8
  IMD_IN/1 -> CAN Pack1/12
  RESET_SIG/1 -> CAN Pack1/14
  SDC_SIG/1 -> CAN Pack1/15
  SDC_SIG_FINAL/1 -> [SDC_SIG_F], CAN Pack1/16
  START_UP_ACTIVE/1 -> CAN Pack1/17
  Knob3/1 -> CAN Pack12/7
  Knob2/1 -> CAN Pack12/6
  Knob1/1 -> CAN Pack12/4
  dash_pot_2/1 -> CAN Pack12/5
  dash_pot_1/1 -> CAN Pack12/3
  dash_pot_3/1 -> CAN Pack1/10
  Regen Switch/1 -> CAN Pack2/5
  NOT/1 -> TSSI_Green_Light_GPIO_25/1
  NOT1/1 -> TSSI_Red_Light_GPIO_27/1
  Brake Light/1 -> NOT13/1
  Buzzer/1 -> NOT3/1
  NOT4/1 -> RTD_LED_GPIO_29/1
  NOT5/1 -> inverter_enable_GPIO_26/1
  NOT6/1 -> Cooling_1_MCU_GPIO_11/1
  NOT7/1 -> Cooling_3_MCU_GPIO_14/1
  NOT8/1 -> Cooling_2_MCU_GPIO_10/1
  NOT9/1 -> TC_LED_1_GPIO_4/1
  NOT10/1 -> TC_LED_2_GPIO_3/1
  NOT11/1 -> TC_LED_3_GPIO_2/1
  NOT12/1 -> TC_LED_4_GPIO_1/1
  Demux/5 -> NOT2/1
  NOT14/1 -> TC_LED_ON_GPIO_5/1
  NOT2/1 -> TC_LED_5_GPIO_0/1
  NOT3/1 -> BUZZER_GPIO_105/1
  NOT13/1 -> brake_light_mcu_GPIO_104/1
  CAN Pack/1 -> Rate Transition4/1
  Rate Transition4/1 -> CAN Transmit/1
  NOT15/1 -> Discharge_CTRL_GPIO_32/1
  Driver Torque Switch/1 -> Rate Transition12/1
  Rate Transition12/1 -> CAN Pack2/2
  Driver_Torque_Switch/1 -> CAN Pack1/11
  MCU Input Control/1 -> CAN Pack1/13
  Digital Clock/1 -> Hit Crossing3/1, MATLAB Function/1(t)
  Hit Crossing/1 -> MATLAB Function/3(sdc_low)
  [SDC_SIG_F] -> Hit Crossing2/1, Hit Crossing/1
  Rate Transition3/1 -> eCAN Transmit1/1
  Hit Crossing2/1 -> MATLAB Function/4(sdc_high)
  Hit Crossing3/1 -> MATLAB Function/2(t_hit)
  DC Bus Voltage/1 -> Less Than/1
  Constant/1 -> Less Than/2
  Less Than/1 -> rtm_GPIO_130/1

== system main/In Signals/Function-Call Subsystem1 ==
  In1 : Inport
  function : TriggerPort  TriggerType=function-call  VariantControl=(inherit)
  CAN Unpack : canmsglib/CAN Unpack  CANdbFile=C:\Users\levin\OneDrive\Documents\GitHub\EV26-Software\CAN\EV26.dbc  MsgList=M168_Flux_ID_IQ_Info  MsgName=M168_Flux_ID_IQ_Info  MsgIDType=Standard (11-bit identifier)  MsgIdentifier=168  MsgLength=8  SignalInfo={'INV_Id','32','16','LE','signed','Standard','0','0.1','0','-3276.8','3276.7';'INV_Iq','48','16','LE','signed','Standard','0','0.1','0','-3276.8','3276.7';'INV_Vd_ff','0','16','LE','signed','Standard','0','0.1','0','-3276.7','3276.7';'INV_Vq_ff','16','16','LE','signed','Standard','0','0.1','0','-3276.7','3276.7'}  IDPort=off  TimestampPort=off  ErrorPort=off  RemotePort=off  LengthPort=off  StatusPort=off  ApplyMinMax=off
      settings: DataFormat=CANdb specified signals
  INV_Id : Outport
  INV_Iq : Outport  Port=2
  wires:
  In1/1 -> CAN Unpack/1
  CAN Unpack/1 -> INV_Id/1
  CAN Unpack/2 -> INV_Iq/1

== system main/In Signals/Function-Call Subsystem10 ==
  In1 : Inport
  function : TriggerPort  TriggerType=function-call  VariantControl=(inherit)
  CAN Unpack : canmsglib/CAN Unpack  CANdbFile=C:\Users\Columbia\Documents\GitHub\EV26-Software\CAN\EV26.dbc  MsgList=(none)  MsgName=M170_Internal_States  MsgIDType=Standard (11-bit identifier)  MsgIdentifier=170  MsgLength=8  SignalInfo={'INV_BMS_Active','57','1','LE','unsigned','Standard','0','1','0','0','1';'INV_BMS_Torque_Limiting','58','1','LE','unsigned','Standard','0','1','0','0','1';'INV_Burst_Model_Mode','49','1','LE','unsigned','Standard','0','1','0','0','1';'INV_Direction_Command','56','1','LE','unsigned','Standard','0','1','0','0','1';'INV_Inverter_Command_Mode','40','1','LE','unsigned','Standard','0','1','0','0','1';'INV_Inverter_Discharge_State','37','3','LE','unsigned','Standard','0','1','0','0','7';'INV_Inverter_Enable_Lockout','55','1','LE','unsigned','Standard','0','1','0','0','1';'INV_Inverter_Enable_State','48','1','LE','unsigned','Standard','0','1','0','0','1';'INV_Inverter_Run_Mode','32','1','LE','unsigned','Standard','0','1','0','0','1';'INV_Inverter_State','16','8','LE','unsigned','Standard','0','1','0','0','255';'INV_Key_Switch_Start_Status','54','1','LE','unsigned','Standard','0','1','0','0','1';'INV_Limit_Coolant_Derating','62','1','LE','unsigned','Standard','0','1','0','0','1';'INV_Limit_Hot_Spot','60','1','LE','unsigned','Standard','0','1','0','0','1';'INV_Limit_Max_Speed','59','1','LE','unsigned','Standard','0','1','0','0','1';'INV_Limit_Stall_Burst_Model','63','1','LE','unsigned','Standard','0','1','0','0','1';'INV_Low_Speed_Limiting','61','1','LE','unsigned','Standard','0','1','0','0','1';'INV_PWM_Frequency','8','8','LE','unsigned','Standard','0','1','0','0','255';'INV_Relay_1_Status','24','1','LE','unsigned','Standard','0','1','0','0','1';'INV_Relay_2_Status','25','1','LE','unsigned','Standard','0','1','0','0','1';'INV_Relay_3_Status','26','1','LE','unsigned','Standard','0','1','0','0','1';'INV_Relay_4_Status','27','1','LE','unsigned','Standard','0','1','0','0','1';'INV_Relay_5_Status','28','1','LE','unsigned','Standard','0','1','0','0','1';'INV_Relay_6_Status','29','1','LE','unsigned','Standard','0','1','0','0','1';'INV_Rolling_Counter','44','4','LE','unsigned','Standard','0','1','0','0','15';'INV_Self_Sensing_Assist_Enable','33','1','LE','unsigned','Standard','0','1','0','0','1';'INV_VSM_State','0','8','LE','unsigned','Standard','0','1','0','0','15'}  IDPort=off  TimestampPort=off  ErrorPort=off  RemotePort=off  LengthPort=off  StatusPort=off  ApplyMinMax=off
      settings: DataFormat=CANdb specified signals
  inv_en : Outport  OutDataTypeStr=uint8
  wires:
  In1/1 -> CAN Unpack/1
  CAN Unpack/8 -> inv_en/1

== system main/In Signals/Function-Call Subsystem11 ==
  In1 : Inport
  function : TriggerPort  TriggerType=function-call  VariantControl=(inherit)
  CAN Unpack1 : canmsglib/CAN Unpack  CANdbFile=C:\Users\levin\OneDrive\Documents\GitHub\EV26-Software\CAN\EV26.dbc  MsgList=M002_TS_State  MsgName=M002_TS_State  MsgIDType=Standard (11-bit identifier)  MsgIdentifier=2  MsgLength=7  SignalInfo={'TB_BSM_Discharge','32','1','LE','unsigned','Standard','0','1','0','0','1';'TB_IR_Minus_Aux','48','1','LE','unsigned','Standard','0','1','0','0','1';'TB_IR_Minus_Enable','24','1','LE','unsigned','Standard','0','1','0','0','1';'TB_IR_Plus_Aux','40','1','LE','unsigned','Standard','0','1','0','0','1';'TB_IR_Plus_Enable','16','1','LE','unsigned','Standard','0','1','0','0','1';'TB_PC_Enable','8','1','LE','unsigned','Standard','0','1','0','0','1';'TB_TS_State','0','8','LE','signed','Standard','0','1','0','-Inf','Inf'}  IDPort=off  TimestampPort=off  ErrorPort=off  RemotePort=off  LengthPort=off  StatusPort=off  ApplyMinMax=off
      settings: DataFormat=CANdb specified signals
  ts_state : Outport  OutDataTypeStr=int8
  bsm_discharge : Outport  Port=2
  wires:
  In1/1 -> CAN Unpack1/1
  CAN Unpack1/7 -> ts_state/1
  CAN Unpack1/1 -> bsm_discharge/1

== system main/In Signals/Function-Call Subsystem2 ==
  In1 : Inport
  function : TriggerPort  TriggerType=function-call  VariantControl=(inherit)
  CAN Unpack : canmsglib/CAN Unpack  CANdbFile=C:\Users\levin\OneDrive\Documents\GitHub\EV26-Software\CAN\EV26.dbc  MsgList=M166_Current_Info  MsgName=M166_Current_Info  MsgIDType=Standard (11-bit identifier)  MsgIdentifier=166  MsgLength=8  SignalInfo={'INV_DC_Bus_Current','48','16','LE','signed','Standard','0','0.1','0','-3276.8','3276.7';'INV_Phase_A_Current','0','16','LE','signed','Standard','0','0.1','0','-3276.8','3276.7';'INV_Phase_B_Current','16','16','LE','signed','Standard','0','0.1','0','-3276.8','3276.7';'INV_Phase_C_Current','32','16','LE','signed','Standard','0','0.1','0','-3276.8','3276.7'}  IDPort=off  TimestampPort=off  ErrorPort=off  RemotePort=off  LengthPort=off  StatusPort=off  ApplyMinMax=off
      settings: DataFormat=CANdb specified signals
  DC Bus Current : Outport
  wires:
  In1/1 -> CAN Unpack/1
  CAN Unpack/1 -> DC Bus Current/1

== system main/In Signals/Function-Call Subsystem3 ==
  In1 : Inport
  function : TriggerPort  TriggerType=function-call  VariantControl=(inherit)
  CAN Unpack : canmsglib/CAN Unpack  CANdbFile=C:\Users\levin\OneDrive\Documents\GitHub\EV26-Software\CAN\EV26.dbc  MsgList=M237_BMS_Stats  MsgName=M237_BMS_Stats  MsgIDType=Standard (11-bit identifier)  MsgIdentifier=237  MsgLength=8  SignalInfo={'BMS_Max_Temp','16','8','LE','unsigned','Standard','0','0.25','0','0','63.75';'BMS_Max_Temp_Idx','48','8','LE','unsigned','Standard','0','1','0','-Inf','Inf';'BMS_Max_Volt_Idx','32','8','LE','unsigned','Standard','0','1','0','-Inf','Inf';'BMS_Max_Voltage','0','8','LE','unsigned','Standard','0','0.01','1.8','1.8','4.35';'BMS_Min_Temp','24','8','LE','unsigned','Standard','0','0.25','0','0','63.75';'BMS_Min_Temp_Idx','56','8','LE','unsigned','Standard','0','1','0','-Inf','Inf';'BMS_Min_Volt_Idx','40','8','LE','unsigned','Standard','0','1','0','-Inf','Inf';'BMS_Min_Voltage','8','8','LE','unsigned','Standard','0','0.01','1.8','1.8','4.35'}  IDPort=off  TimestampPort=off  ErrorPort=off  RemotePort=off  LengthPort=off  StatusPort=off  ApplyMinMax=off
      settings: DataFormat=CANdb specified signals
  BMS Min Voltage : Outport
  wires:
  In1/1 -> CAN Unpack/1
  CAN Unpack/8 -> BMS Min Voltage/1

== system main/In Signals/Function-Call Subsystem6 ==
  In2 : Inport
  In1 : Inport  Port=2
  function : TriggerPort  TriggerType=function-call  VariantControl=(inherit)
  CAN Unpack : canmsglib/CAN Unpack  CANdbFile=C:\Users\Columbia\Documents\GitHub\EV26-Software\CAN\EV26.dbc  MsgList=(none)  MsgName=M051_Wheel_Speeds  MsgIDType=Standard (11-bit identifier)  MsgIdentifier=51  MsgLength=8  SignalInfo={'SEN_WSS_FL','0','16','LE','unsigned','Standard','0','0.1','0','0','6553.5';'SEN_WSS_FR','16','16','LE','unsigned','Standard','0','0.1','0','0','163.8375';'SEN_WSS_RL','32','16','LE','unsigned','Standard','0','0.1','0','0','6553.5';'SEN_WSS_RR','48','16','LE','unsigned','Standard','0','0.1','0','0','6553.5'}  IDPort=off  TimestampPort=off  ErrorPort=off  RemotePort=off  LengthPort=off  StatusPort=off  ApplyMinMax=off
      settings: DataFormat=CANdb specified signals
  FL : Outport  OutDataTypeStr=double
  FR : Outport  Port=2  OutDataTypeStr=double
  RL : Outport  Port=3  OutDataTypeStr=double
  RR : Outport  Port=4  OutDataTypeStr=double
  Velocity Timestamp : Outport  Port=5
  wires:
  In1/1 -> CAN Unpack/1
  CAN Unpack/1 -> FL/1
  CAN Unpack/4 -> RR/1
  CAN Unpack/2 -> FR/1
  CAN Unpack/3 -> RL/1
  In2/1 -> Velocity Timestamp/1

== system main/In Signals/Function-Call Subsystem7 ==
  In1 : Inport
  In2 : Inport  Port=2
  function : TriggerPort  TriggerType=function-call  VariantControl=(inherit)
  CAN Unpack : canmsglib/CAN Unpack  CANdbFile=C:\Users\levin\OneDrive\Documents\GitHub\EV26-Software\CAN\EV26.dbc  MsgList=M052_G_Forces  MsgName=M052_G_Forces  MsgIDType=Standard (11-bit identifier)  MsgIdentifier=52  MsgLength=8  SignalInfo={'LV_IMU_Acceleration','48','8','LE','signed','Standard','0','0.1','0','-12.8','12.7';'LV_IMU_Angular_Rate','56','8','LE','signed','Standard','0','1','0','-128','127';'SEN_G_FORCE_X','0','16','LE','signed','Standard','0','0.01','0','-327.68','327.67';'SEN_G_FORCE_Y','16','16','LE','signed','Standard','0','0.01','0','-327.68','327.67';'SEN_G_FORCE_Z','32','16','LE','signed','Standard','0','0.01','0','-327.68','327.67'}  IDPort=off  TimestampPort=off  ErrorPort=off  RemotePort=off  LengthPort=off  StatusPort=off  ApplyMinMax=off
      settings: DataFormat=CANdb specified signals
  Long Accel : Outport  OutDataTypeStr=double
  Accel Report : Outport  Port=2
  Lateral Accel : Outport  Port=3
  wires:
  In1/1 -> CAN Unpack/1
  CAN Unpack/3 -> Long Accel/1
  CAN Unpack/4 -> Lateral Accel/1
  In2/1 -> Accel Report/1

== system main/In Signals/Function-Call Subsystem8 ==
  In1 : Inport
  function : TriggerPort  TriggerType=function-call  VariantControl=(inherit)
  CAN Unpack : canmsglib/CAN Unpack  CANdbFile=C:\Users\willi\Desktop\FSAE\EV26-Software\CAN\EV26.dbc  MsgList=(none)  MsgName=M167_Voltage_Info  MsgIDType=Standard (11-bit identifier)  MsgIdentifier=167  MsgLength=8  SignalInfo={'INV_DC_Bus_Voltage','0','16','LE','signed','Standard','0','0.1','0','-3276.8','3276.7';'INV_Output_Voltage','16','16','LE','signed','Standard','0','0.1','0','-3276.8','3276.7';'INV_VAB_Vd_Voltage','32','16','LE','signed','Standard','0','0.1','0','-3276.8','3276.7';'INV_VBC_Vq_Voltage','48','16','LE','signed','Standard','0','0.1','0','-3276.8','3276.7'}  IDPort=off  TimestampPort=off  ErrorPort=off  RemotePort=off  LengthPort=off  StatusPort=off  ApplyMinMax=off
      settings: DataFormat=CANdb specified signals
  DC_Bus_Voltage : Outport
  wires:
  In1/1 -> CAN Unpack/1
  CAN Unpack/1 -> DC_Bus_Voltage/1

== system main/In Signals/Subsystem1 ==
  In1 : Inport
  function : TriggerPort  TriggerType=function-call  VariantControl=(inherit)
  CAN Unpack : canmsglib/CAN Unpack  CANdbFile=C:\Users\willi\Desktop\FSAE\EV26-Software\CAN\EV26.dbc  MsgList=(none)  MsgName=M165_Motor_Position_Info  MsgIDType=Standard (11-bit identifier)  MsgIdentifier=165  MsgLength=8  SignalInfo={'INV_Delta_Resolver_Filtered','48','16','LE','signed','Standard','0','0.1','0','-3276.8','3276.7';'INV_Electrical_Output_Frequency','32','16','LE','signed','Standard','0','0.1','0','-3276.8','3276.7';'INV_Motor_Angle_Electrical','0','16','LE','unsigned','Standard','0','0.1','0','0','6553.5';'INV_Motor_Speed','16','16','LE','signed','Standard','0','1','0','-32768','32767'}  IDPort=off  TimestampPort=off  ErrorPort=off  RemotePort=off  LengthPort=off  StatusPort=off  ApplyMinMax=off
      settings: LibrarySourceBlock=c2000lib/Target Communication/CAN Unpack  DataFormat=CANdb specified signals
  Out1 : Outport
  wires:
  CAN Unpack/4 -> Out1/1
  In1/1 -> CAN Unpack/1

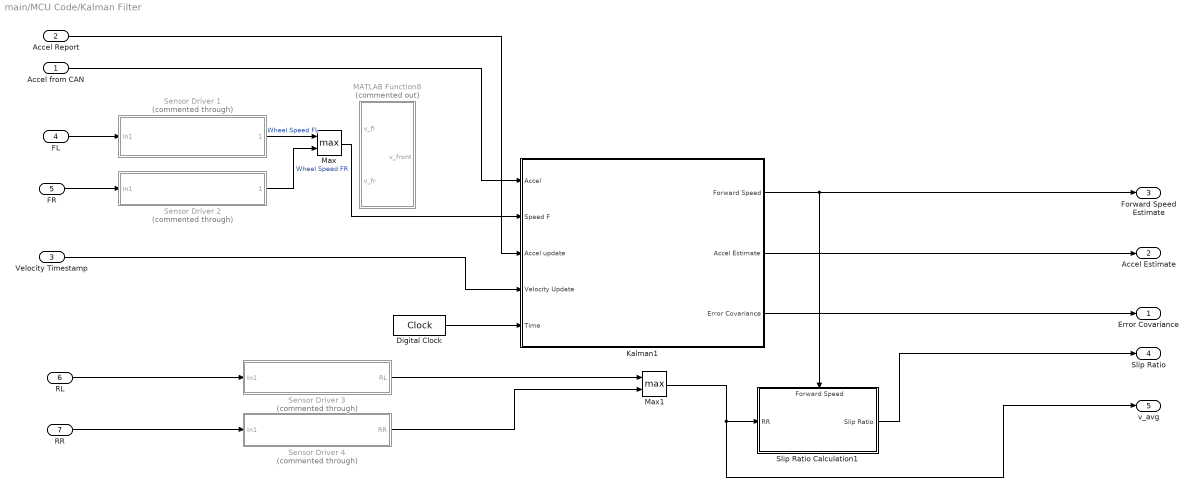
== system main/MCU Code/Kalman Filter ==
  Accel from CAN : Inport
  Accel Report : Inport  Port=2
  Velocity Timestamp : Inport  Port=3
  FL : Inport  Port=4
  FR : Inport  Port=5
  RL : Inport  Port=6
  RR : Inport  Port=7
  Digital Clock : DigitalClock  SampleTime=0.001
  Kalman1 : Subsystem
  MATLAB Function8 : MATLAB Function  Commented=on  TreatAsAtomicUnit=on
  Max : MinMax  Function=max  Inputs=2
  Max1 : MinMax  Function=max  Inputs=2
  Sensor Driver 1 : Subsystem  Commented=through
  Sensor Driver 2 : Subsystem  Commented=through
  Sensor Driver 3 : Subsystem  Commented=through
  Sensor Driver 4 : Subsystem  Commented=through
  Slip Ratio Calculation1 : Subsystem
      settings: PortSchema="{\"entries\":[{\"content\":{\"sides\":[{\"content\":{\"connectorIds\":[\"In1\"]},\"type\":\"ConnectorPlacement.EquallySpacedRectSide\",\"uuid\":\"061c82cd-7e9c-4a72-b965-43235230dad9\"},{\"content\":{\"connectorIds\":[\"Out1\"],\"side\":\"RIGHT\"},\"type\":\"ConnectorPlacement.EquallySpacedRectSide\",\"uuid\":\"899eaa50-1c30-4f77-9d66-a8daefd9f1e3\"},{\"content\":{\"connectorIds\":[\"In2\"],\"side\":\"TOP\"},\"type\":\"ConnectorPlacement.EquallySpacedRectSide\",\"uuid\":\"89c07a25-5c36-4b16-a58e-7fbb1fd4b8e3\"}]},\"type\":\"ConnectorPlacement.EquallySpacedConnector\",\"uuid\":\"4f00da10-bd17-48bb-8760-fc873e4c20ca\"}],\"packageUris\":[\"http://schema.mathworks.com/mf0/Connector/R2020b\"],\"version\":\"1.0\"}"
  Error Covariance : Outport
  Accel Estimate : Outport  Port=2
  Forward Speed Estimate : Outport  Port=3
  Slip Ratio : Outport  Port=4
  v_avg : Outport  Port=5
  wires:
  Kalman1/1(Forward Speed) -> Slip Ratio Calculation1/2(Forward Speed), Forward Speed Estimate/1
  Slip Ratio Calculation1/1(Slip Ratio) -> Slip Ratio/1
  FR/1 -> Sensor Driver 2/1(In1)
  Sensor Driver 4/1(RR) -> Max1/2
  Sensor Driver 2/1(" ") -> Max/2  "Wheel Speed FR"
  RL/1 -> Sensor Driver 3/1(In1)
  Sensor Driver 1/1(" ") -> Max/1  "Wheel Speed FL"
  FL/1 -> Sensor Driver 1/1(In1)
  Sensor Driver 3/1(RL) -> Max1/1
  Accel from CAN/1 -> Kalman1/1(Accel)
  RR/1 -> Sensor Driver 4/1(In1)
  Digital Clock/1 -> Kalman1/5(Time)
  Kalman1/2(Accel Estimate) -> Accel Estimate/1
  Kalman1/3(Error Covariance) -> Error Covariance/1
  Velocity Timestamp/1 -> Kalman1/4(Velocity Update)
  Accel Report/1 -> Kalman1/3(Accel update)
  Max/1 -> Kalman1/2(Speed F)
  Max1/1 -> Slip Ratio Calculation1/1(RR), v_avg/1

== system main/MCU Code/Motec Screen ==
  Screen Button : Inport
  TC Button : Inport  Port=2
  Cast To Boolean : DataTypeConversion  OutDataTypeStr=boolean  SaturateOnIntegerOverflow=off  RndMeth=Floor
  Cast To Double : DataTypeConversion  OutDataTypeStr=double  SaturateOnIntegerOverflow=off  RndMeth=Floor
  Hit Crossing : HitCross  HitCrossingOffset=0.5  HitCrossingDirection=rising
  MATLAB Function : MATLAB Function  TreatAsAtomicUnit=on
  MATLAB Function10 : MATLAB Function  TreatAsAtomicUnit=on
  Screen : Outport
  TC_switch : Outport  Port=2
  wires:
  MATLAB Function10/1(page) -> Screen/1
  Hit Crossing/1 -> MATLAB Function10/1(screen_button)
  TC Button/1 -> MATLAB Function/1(TC_Button)
  Screen Button/1 -> Cast To Double/1
  MATLAB Function/1(TC_switch) -> Cast To Boolean/1
  Cast To Boolean/1 -> TC_switch/1
  Cast To Double/1 -> Hit Crossing/1

== system main/MCU Code/Pedals Curve ==
  u : Inport
  1-D Lookup Table : Lookup_n-D  Commented=on  NumberOfTableDimensions=1  BreakpointsForDimension1=linspace(0,1,100)  TableSource=Input port  Table=linspace(0,1,100).^1.5  InternalRulePriority=Speed  RndMeth=Simplest
      settings: InputPortMap=u0,p221
  1-D Lookup Table1 : Lookup_n-D  Commented=on  NumberOfTableDimensions=1  BreakpointsForDimension1=[1 10]  Table=[1 5.5]  InternalRulePriority=Speed  RndMeth=Simplest
  MATLAB Function : MATLAB Function  Commented=on  TreatAsAtomicUnit=on
  Pedal Curve : Lookup_n-D  NumberOfTableDimensions=1  BreakpointsForDimension1=[0 1]  Table=[0 1]  ExtrapMethod=Clip  UseLastTableValue=on  InternalRulePriority=Speed  RndMeth=Simplest
  ped : Outport
  wires:
  u/1 -> Pedal Curve/1
  MATLAB Function/1(table) -> 1-D Lookup Table/2
  1-D Lookup Table1/1 -> MATLAB Function/1(exp)
  Pedal Curve/1 -> ped/1

== system main/MCU Code/Power Limiting ==
  In1 : Inport
  In2 : Inport  Port=2
  1-D Lookup Table4 : Lookup_n-D  NumberOfTableDimensions=1  BreakpointsForDimension1=[1;10]  Table=[10e3;80e3]  ExtrapMethod=Clip  InternalRulePriority=Speed  RndMeth=Simplest
  Divide : Product  Inputs=*/
  Moving Average : Subsystem
  Saturation2 : Saturate  UpperLimit=inf  LowerLimit=1
  to rad/s : Gain  Gain=2*pi/60
  Out1 : Outport
  wires:
  Divide/1 -> Out1/1
  to rad/s/1 -> Moving Average/1(In1)
  Moving Average/1(Out1) -> Saturation2/1
  Saturation2/1 -> Divide/2
  1-D Lookup Table4/1 -> Divide/1
  In1/1 -> 1-D Lookup Table4/1
  In2/1 -> to rad/s/1
